simulink model "pid20180920"  (R2018b)
settings: Solver=ode3  StartTime=0.0  StopTime=5  FixedStep=0.02  RelTol=1e-3
settings Model: Creator=Think  LastModifiedBy=think
settings DataIOCC: LimitDataPoints=on  SaveFormat=Array
settings OptimizationCC: BlockReduction=off  BooleanDataType=off  LifeSpan=inf
settings DebuggingCC: SaveWithParameterizedLinksMsg=none  UnderspecifiedInitializationDetection=Classic  MergeDetectMultiDrivingBlocksExec=none  SignalResolutionControl=TryResolveAllWithWarning  SFUnexpectedBacktrackingDiag=warning  SFNoUnconditionalDefaultTransitionDiag=warning  SFExecutionAtInitializationDiag=none
settings HardwareCC: ProdBitPerPointer=32  ProdBitPerSizeT=32  ProdBitPerPtrDiffT=32  ProdLargestAtomicFloat=None  ProdIntDivRoundTo=Undefined  ProdEndianess=Unspecified  ProdWordSize=32  ProdHWDeviceType=32-bit Generic  TargetUnknown=on
settings ModelReferenceCC: PropagateSignalLabelsOutOfModel=off
settings SFSimCC: SimUseLocalCustomCode=off
settings RTWCC: RTWUseLocalCustomCode=off
settings CodeAppCC: StateflowObjectComments=on
settings GRTTargetCC: TargetLangStandard=C89/C90 (ANSI)  GeneratePreprocessorConditionals=Disable all
settings ConfigComp: CovMetricSettings=dw  CovHtmlReporting=on  CovSaveCumulativeToWorkspaceVar=on  CovSaveSingleToWorkspaceVar=on  CovExternalEMLEnable=off  CovSFcnEnable=off

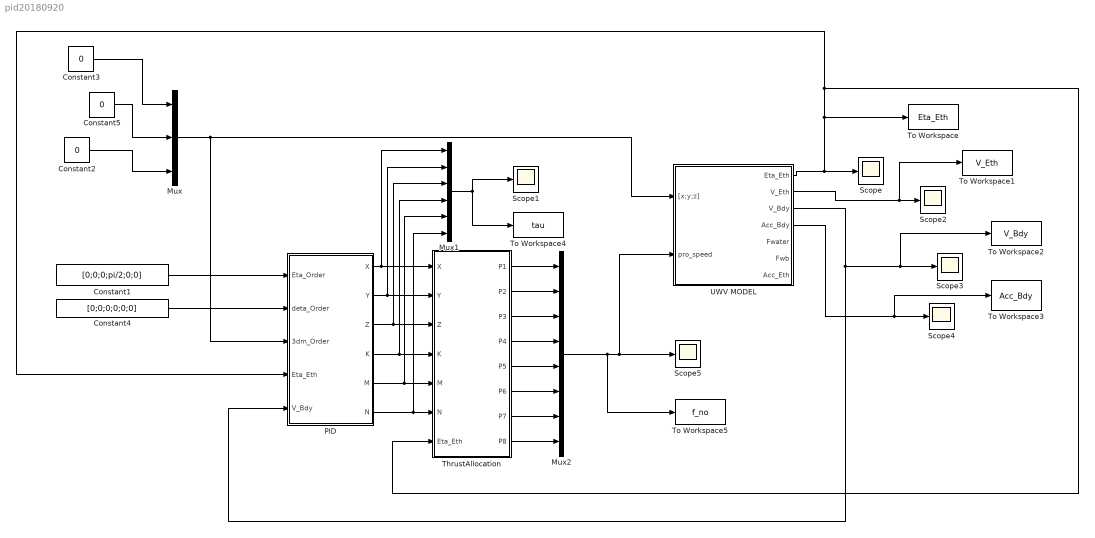
== system pid20180920 ==
  Constant1 : Constant  Value=[0;0;0;pi/2;0;0]
  Constant2 : Constant  Value=0
  Constant3 : Constant  Value=0
  Constant4 : Constant  Value=[0;0;0;0;0;0]
  Constant5 : Constant  Value=0
  Mux : Mux  Inputs=3
  Mux1 : Mux  Inputs=6
  Mux2 : Mux  Inputs=8
  PID : Subsystem
  Scope{,1..5} (6 alike) : Scope
  ThrustAllocation : Subsystem
  To Workspace : ToWorkspace  VariableName=Eta_Eth  SaveFormat=Timeseries  SampleTime=-1
  To Workspace1 : ToWorkspace  VariableName=V_Eth  SaveFormat=Timeseries  SampleTime=-1
  To Workspace2 : ToWorkspace  VariableName=V_Bdy  SaveFormat=Timeseries  SampleTime=-1
  To Workspace3 : ToWorkspace  VariableName=Acc_Bdy  SaveFormat=Timeseries  SampleTime=-1
  To Workspace4 : ToWorkspace  VariableName=tau  SaveFormat=Timeseries  SampleTime=-1
  To Workspace5 : ToWorkspace  VariableName=f_no  SaveFormat=Timeseries  SampleTime=-1
  UWV MODEL : Subsystem
  wires:
  Mux/1 -> PID/3(3dm_Order), UWV MODEL/1("[x;y;z]")
  UWV MODEL/2(V_Eth) -> To Workspace1/1, Scope2/1
  UWV MODEL/3(V_Bdy) -> PID/5(V_Bdy), To Workspace2/1, Scope3/1
  UWV MODEL/4(Acc_Bdy) -> To Workspace3/1, Scope4/1
  Constant2/1 -> Mux/3
  Constant3/1 -> Mux/1
  ThrustAllocation/1(P1) -> Mux2/1
  ThrustAllocation/2(P2) -> Mux2/2
  ThrustAllocation/3(P3) -> Mux2/3
  ThrustAllocation/4(P4) -> Mux2/4
  ThrustAllocation/5(P5) -> Mux2/5
  ThrustAllocation/6(P6) -> Mux2/6
  ThrustAllocation/7(P7) -> Mux2/7
  ThrustAllocation/8(P8) -> Mux2/8
  UWV MODEL/1(Eta_Eth) -> PID/4(Eta_Eth), ThrustAllocation/7(Eta_Eth), To Workspace/1, Scope/1
  Constant1/1 -> PID/1(Eta_Order)
  Constant4/1 -> PID/2(deta_Order)
  Mux2/1 -> To Workspace5/1, UWV MODEL/2(pro_speed), Scope5/1
  PID/1(X) -> Mux1/1, ThrustAllocation/1(X)
  PID/2(Y) -> Mux1/2, ThrustAllocation/2(Y)
  PID/3(Z) -> Mux1/3, ThrustAllocation/3(Z)
  PID/4(K) -> Mux1/4, ThrustAllocation/4(K)
  PID/5(M) -> Mux1/5, ThrustAllocation/5(M)
  PID/6(N) -> Mux1/6, ThrustAllocation/6(N)
  Mux1/1 -> To Workspace4/1, Scope1/1
  Constant5/1 -> Mux/2

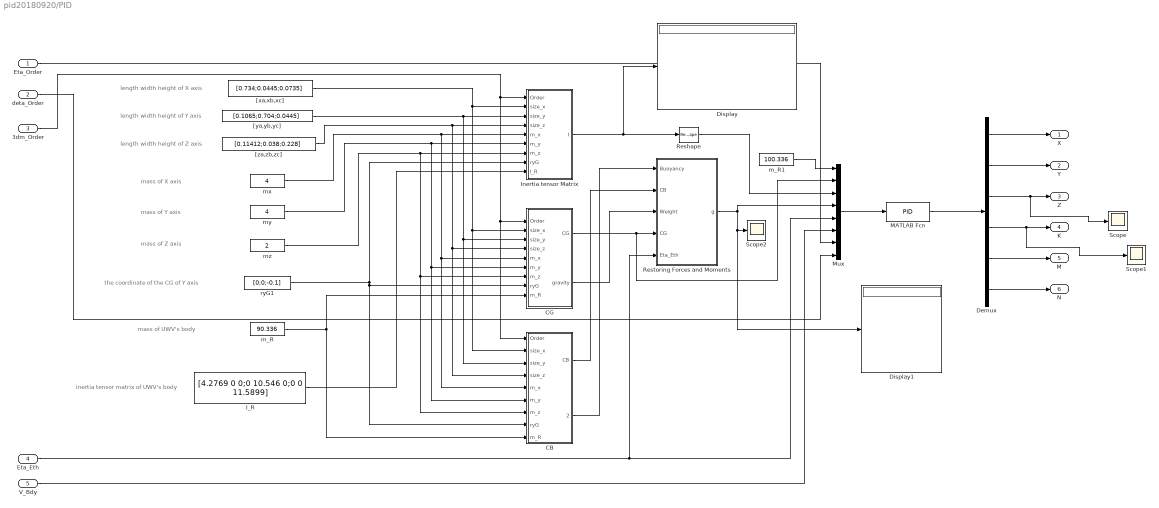
== system pid20180920/PID ==
  note: mass of Z axis
  note: mass of X axis
  note: mass of Y axis
  note: length width height of Y axis
  note: length width height of Z axis
  note: length width height of X axis
  note: the coordinate of the CG of Y axis
  note: mass of UWV's body
  note: inertia tensor matrix of UWV's body
  Eta_Order : Inport
  deta_Order : Inport  Port=2
  3dm_Order : Inport  Port=3
  Eta_Eth : Inport  Port=4
  V_Bdy : Inport  Port=5
  CB : Subsystem
  CG : Subsystem
  Demux : Demux  Outputs=6
  Display : Display
  Display1 : Display
  I_R : Constant  Value=[4.2769 0 0;0 10.546 0;0 0 11.5899]
  Inertia tensor Matrix : Subsystem
  MATLAB Fcn : MATLABFcn  MATLABFcn=PID  OutputDimensions=6  Output1D=off
  Mux : Mux  Inputs=8
  Reshape : Reshape
  Restoring Forces and Moments : Subsystem
  Scope : Scope
  Scope1 : Scope
  Scope2 : Scope
  "[xa,xb,xc]" : Constant  Value=[0.734;0.0445;0.0735]
  "[ya,yb,yc]" : Constant  Value=[0.1065;0.704;0.0445]
  "[za,zb,zc]" : Constant  Value=[0.11412;0.038;0.228]
  m_R : Constant  Value=90.336
  m_R1 : Constant  Value=100.336
  mx : Constant  Value=4
  my : Constant  Value=4
  mz : Constant  Value=2
  ryG1 : Constant  Value=[0;0;-0.1]
  X : Outport
  Y : Outport  Port=2
  Z : Outport  Port=3
  K : Outport  Port=4
  M : Outport  Port=5
  N : Outport  Port=6
  wires:
  CG/1(CG) -> Mux/2, Restoring Forces and Moments/4(CG)
  CG/2(gravity) -> Restoring Forces and Moments/3(Weight)
  CB/1(CB) -> Restoring Forces and Moments/2(CB)
  CB/2(Buoyancy) -> Restoring Forces and Moments/1(Buoyancy)
  Mux/1 -> MATLAB Fcn/1
  Reshape/1 -> Mux/3
  Eta_Eth/1 -> Restoring Forces and Moments/5(Eta_Eth), Mux/5
  V_Bdy/1 -> Mux/6
  Eta_Order/1 -> Mux/7
  "[xa,xb,xc]"/1 -> CB/2(size_x), CG/2(size_x), Inertia tensor Matrix/2(size_x)
  "[ya,yb,yc]"/1 -> CB/3(size_y), CG/3(size_y), Inertia tensor Matrix/3(size_y)
  "[za,zb,zc]"/1 -> CB/4(size_z), CG/4(size_z), Inertia tensor Matrix/4(size_z)
  mx/1 -> CB/5(m_x), CG/5(m_x), Inertia tensor Matrix/5(m_x)
  my/1 -> CB/6(m_y), CG/6(m_y), Inertia tensor Matrix/6(m_y)
  mz/1 -> CB/7(m_z), CG/7(m_z), Inertia tensor Matrix/7(m_z)
  ryG1/1 -> CB/8(ryG), CG/8(ryG), Inertia tensor Matrix/8(ryG)
  m_R/1 -> CG/9(m_R), CB/9(m_R)
  I_R/1 -> Inertia tensor Matrix/9(I_R)
  m_R1/1 -> Mux/1
  MATLAB Fcn/1 -> Demux/1
  Demux/1 -> X/1
  Demux/2 -> Y/1
  Demux/3 -> Scope/1, Z/1
  Demux/4 -> Scope1/1, K/1
  Demux/5 -> M/1
  Demux/6 -> N/1
  deta_Order/1 -> Mux/8
  Inertia tensor Matrix/1(I) -> Display/1, Reshape/1
  3dm_Order/1 -> CB/1(Order), CG/1(Order), Inertia tensor Matrix/1(Order)
  Restoring Forces and Moments/1(g) -> Scope2/1, Display1/1, Mux/4

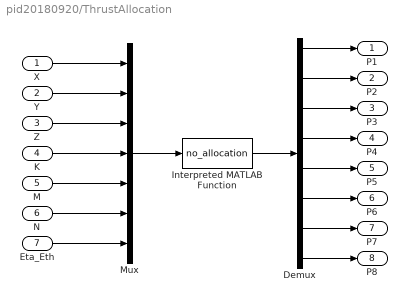
== system pid20180920/ThrustAllocation ==
  X : Inport
  Y : Inport  Port=2
  Z : Inport  Port=3
  K : Inport  Port=4
  M : Inport  Port=5
  N : Inport  Port=6
  Eta_Eth : Inport  Port=7
  Demux : Demux  Outputs=8
  Interpreted MATLAB Function : MATLABFcn  MATLABFcn=no_allocation  OutputDimensions=8
  Mux : Mux  Inputs=7
  P1 : Outport
  P2 : Outport  Port=2
  P3 : Outport  Port=3
  P4 : Outport  Port=4
  P5 : Outport  Port=5
  P6 : Outport  Port=6
  P7 : Outport  Port=7
  P8 : Outport  Port=8
  wires:
  Mux/1 -> Interpreted MATLAB Function/1
  X/1 -> Mux/1
  Y/1 -> Mux/2
  Z/1 -> Mux/3
  K/1 -> Mux/4
  M/1 -> Mux/5
  N/1 -> Mux/6
  Eta_Eth/1 -> Mux/7
  Interpreted MATLAB Function/1 -> Demux/1
  Demux/8 -> P8/1
  Demux/1 -> P1/1
  Demux/2 -> P2/1
  Demux/3 -> P3/1
  Demux/4 -> P4/1
  Demux/5 -> P5/1
  Demux/6 -> P6/1
  Demux/7 -> P7/1

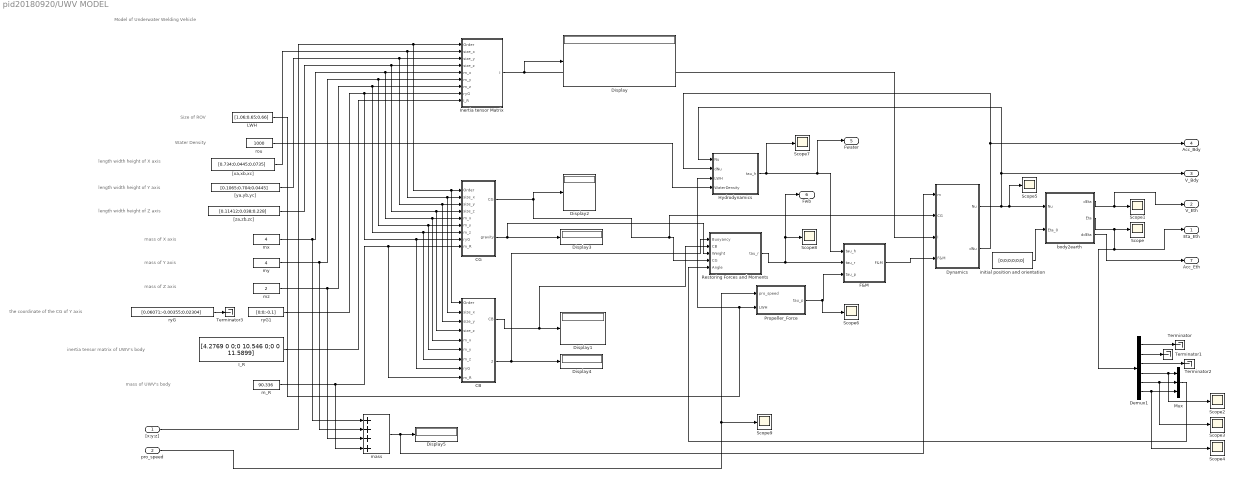
== system pid20180920/UWV MODEL ==
  note: mass of Z axis
  note: length width height of Y axis
  note: the coordinate of the CG of Y axis
  note: length width height of Z axis
  note: mass of UWV's body
  note: mass of X axis
  note: Water Density
  note: length width height of X axis
  note: mass of Y axis
  note: Size of ROV
  note: inertia tensor matrix of UWV's body
  note: Model of Underwater Welding Vehicle
  "[x;y;z]" : Inport
  pro_speed : Inport  Port=2
  CB : Subsystem
  CG : Subsystem
  Demux1 : Demux  Outputs=6
  Display{,1..5} (6 alike) : Display
  Dynamics : Subsystem
  F&M : Subsystem
  Hydrodynamics : Subsystem
  I_R : Constant  Value=[4.2769 0 0;0 10.546 0;0 0 11.5899]
  Inertia tensor Matrix : Subsystem
  LWH : Constant  Value=[1.06;0.65;0.66]
  Mux : Mux  Inputs=3
  Propeller_Force : Subsystem
  Restoring Forces and Moments : Subsystem
  Scope{,1..9} (10 alike) : Scope
  Terminator{,1..3} (4 alike) : Terminator
  "[xa,xb,xc]" : Constant  Value=[0.734;0.0445;0.0735]
  "[ya,yb,yc]" : Constant  Value=[0.1065;0.704;0.0445]
  "[za,zb,zc]" : Constant  Value=[0.11412;0.038;0.228]
  "body2earth " : Subsystem
  initial position and orientation : Constant  Value=[0;0;0;0;0;0]
  m_R : Constant  Value=90.336
  mass : Sum  Inputs=++++
      mask Display:
      | port_label('input',1,'m_x')
      | port_label('input',2,'m_y')
      | port_label('input',3,'m_z')
      | port_label('input',4,'m_R')
      | port_label('output',1,'m')
  mx : Constant  Value=4
  my : Constant  Value=4
  mz : Constant  Value=2
  rou : Constant  Value=1000
  ryG : Constant  Value=[0.06071;-0.00355;0.02304]
  ryG1 : Constant  Value=[0;0;-0.1]
  Eta_Eth : Outport
  V_Eth : Outport  Port=2
  V_Bdy : Outport  Port=3
  Acc_Bdy : Outport  Port=4
  Fwater : Outport  Port=5
  Fwb : Outport  Port=6
  Acc_Eth : Outport  Port=7
  wires:
  Dynamics/2(dNu) -> Acc_Bdy/1, Hydrodynamics/2(dNu)
  rou/1 -> Hydrodynamics/4(WaterDensity)
  mass/1 -> Dynamics/1(m), Display5/1
  Inertia tensor Matrix/1(I) -> Dynamics/3(I), Display/1
  F&M/1(F&M) -> Dynamics/4(F&M)
  Dynamics/1(Nu) -> V_Bdy/1, Hydrodynamics/1(Nu), Scope5/1, "body2earth "/1(Nu)
  initial position and orientation/1 -> "body2earth "/2(Eta_0)
  "[xa,xb,xc]"/1 -> Inertia tensor Matrix/2(size_x), CB/2(size_x), CG/2(size_x)
  m_R/1 -> mass/4, CB/9(m_R), CG/9(m_R)
  mz/1 -> mass/3, CB/7(m_z), CG/7(m_z), Inertia tensor Matrix/7(m_z)
  mx/1 -> mass/1, CB/5(m_x), CG/5(m_x), Inertia tensor Matrix/5(m_x)
  I_R/1 -> Inertia tensor Matrix/9(I_R)
  my/1 -> mass/2, CB/6(m_y), CG/6(m_y), Inertia tensor Matrix/6(m_y)
  "[ya,yb,yc]"/1 -> CB/3(size_y), CG/3(size_y), Inertia tensor Matrix/3(size_y)
  "[x;y;z]"/1 -> Inertia tensor Matrix/1(Order), CB/1(Order), CG/1(Order)
  ryG1/1 -> CB/8(ryG), CG/8(ryG), Inertia tensor Matrix/8(ryG)
  "[za,zb,zc]"/1 -> CB/4(size_z), CG/4(size_z), Inertia tensor Matrix/4(size_z)
  "body2earth "/1(dEta) -> V_Eth/1, Scope1/1
  Restoring Forces and Moments/1(tau_r) -> Fwb/1, Scope8/1, F&M/2(tau_r)
  LWH/1 -> Hydrodynamics/3(LWH), Propeller_Force/2(LWH)
  Demux1/2 -> Terminator1/1
  Demux1/4 -> Scope2/1, Mux/1
  "body2earth "/2(Eta) -> Eta_Eth/1, Demux1/1, Scope/1
  Demux1/1 -> Terminator/1
  Demux1/6 -> Scope4/1, Mux/3
  Demux1/3 -> Terminator2/1
  Demux1/5 -> Scope3/1, Mux/2
  Propeller_Force/1(tau_p) -> Scope6/1, F&M/3(tau_p)
  CG/2(gravity) -> Restoring Forces and Moments/3(Weight), Display3/1
  CB/2(Buoyancy) -> Restoring Forces and Moments/1(Buoyancy), Display4/1
  CG/1(CG) -> Dynamics/2(CG), Restoring Forces and Moments/4(CG), Display2/1
  Mux/1 -> Restoring Forces and Moments/5(Angle)
  ryG/1 -> Terminator3/1
  pro_speed/1 -> Scope9/1, Propeller_Force/1(pro_speed)
  CB/1(CB) -> Restoring Forces and Moments/2(CB), Display1/1
  Hydrodynamics/1(tau_h) -> F&M/1(tau_h), Fwater/1, Scope7/1
  "body2earth "/3(ddEta) -> Acc_Eth/1

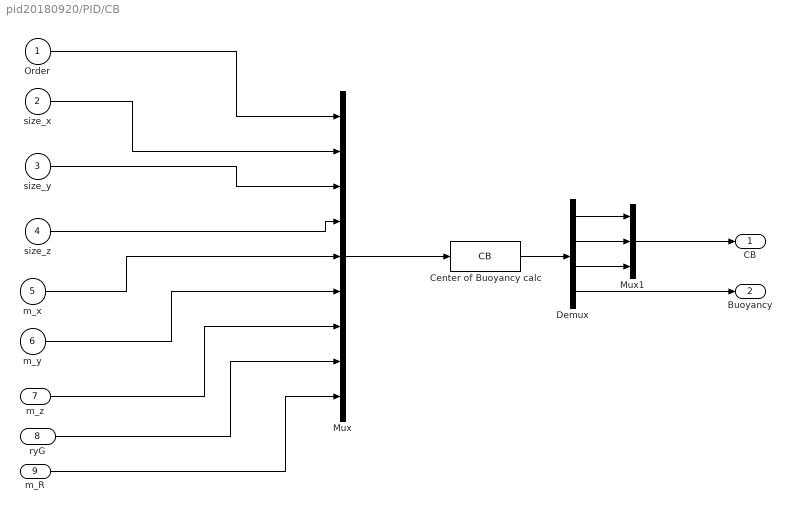
== system pid20180920/PID/CB ==
  Order : Inport
  size_x : Inport  Port=2
  size_y : Inport  Port=3
  size_z : Inport  Port=4
  m_x : Inport  Port=5
  m_y : Inport  Port=6
  m_z : Inport  Port=7
  ryG : Inport  Port=8
  m_R : Inport  Port=9
  Center of Buoyancy calc : MATLABFcn  MATLABFcn=CB  Output1D=off
  Demux : Demux
  Mux : Mux  Inputs=9
  Mux1 : Mux  Inputs=3
  CB : Outport
  Buoyancy : Outport  Port=2
  wires:
  m_x/1 -> Mux/5
  m_y/1 -> Mux/6
  size_x/1 -> Mux/2
  ryG/1 -> Mux/8
  size_z/1 -> Mux/4
  Order/1 -> Mux/1
  size_y/1 -> Mux/3
  m_R/1 -> Mux/9
  m_z/1 -> Mux/7
  Mux/1 -> Center of Buoyancy calc/1
  Center of Buoyancy calc/1 -> Demux/1
  Demux/1 -> Mux1/1
  Demux/2 -> Mux1/2
  Demux/3 -> Mux1/3
  Demux/4 -> Buoyancy/1
  Mux1/1 -> CB/1

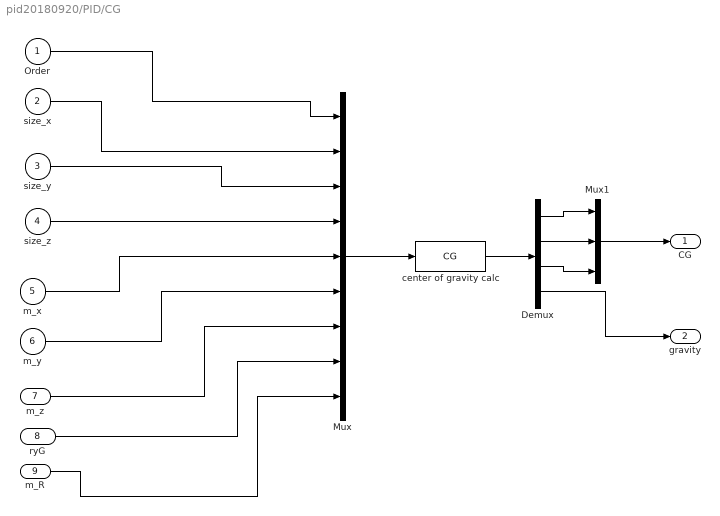
== system pid20180920/PID/CG ==
  Order : Inport
  size_x : Inport  Port=2
  size_y : Inport  Port=3
  size_z : Inport  Port=4
  m_x : Inport  Port=5
  m_y : Inport  Port=6
  m_z : Inport  Port=7
  ryG : Inport  Port=8
  m_R : Inport  Port=9
  Demux : Demux
  Mux : Mux  Inputs=9
  Mux1 : Mux  Inputs=3
  center of gravity calc : MATLABFcn  MATLABFcn=CG  Output1D=off
  CG : Outport
  gravity : Outport  Port=2
  wires:
  Mux/1 -> center of gravity calc/1
  center of gravity calc/1 -> Demux/1
  Demux/1 -> Mux1/1
  Demux/2 -> Mux1/2
  Mux1/1 -> CG/1
  Demux/4 -> gravity/1
  Order/1 -> Mux/1
  size_x/1 -> Mux/2
  size_y/1 -> Mux/3
  size_z/1 -> Mux/4
  m_x/1 -> Mux/5
  m_y/1 -> Mux/6
  ryG/1 -> Mux/8
  m_R/1 -> Mux/9
  m_z/1 -> Mux/7
  Demux/3 -> Mux1/3

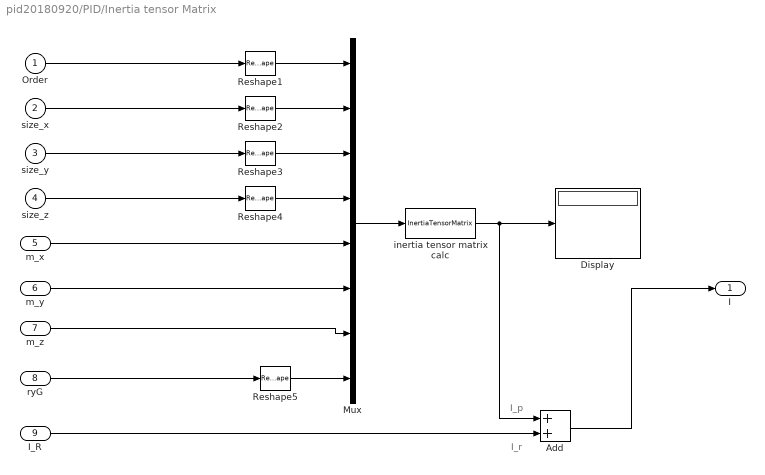
== system pid20180920/PID/Inertia tensor Matrix ==
  note: I_r
  note: I_p
  Order : Inport
  size_x : Inport  Port=2
  size_y : Inport  Port=3
  size_z : Inport  Port=4
  m_x : Inport  Port=5
  m_y : Inport  Port=6
  m_z : Inport  Port=7
  ryG : Inport  Port=8
  I_R : Inport  Port=9
  Add : Sum
  Display : Display
  Mux : Mux  Inputs=8
  Reshape{1..5} (5 alike) : Reshape  OutputDimensions=9
  inertia tensor matrix calc : MATLABFcn  MATLABFcn=InertiaTensorMatrix  Output1D=off
  I : Outport
  wires:
  inertia tensor matrix calc/1 -> Display/1, Add/1
  Mux/1 -> inertia tensor matrix calc/1
  m_z/1 -> Mux/7
  size_z/1 -> Reshape4/1
  m_x/1 -> Mux/5
  Order/1 -> Reshape1/1
  m_y/1 -> Mux/6
  size_x/1 -> Reshape2/1
  size_y/1 -> Reshape3/1
  ryG/1 -> Reshape5/1
  Add/1 -> I/1
  I_R/1 -> Add/2
  Reshape1/1 -> Mux/1
  Reshape2/1 -> Mux/2
  Reshape3/1 -> Mux/3
  Reshape4/1 -> Mux/4
  Reshape5/1 -> Mux/8

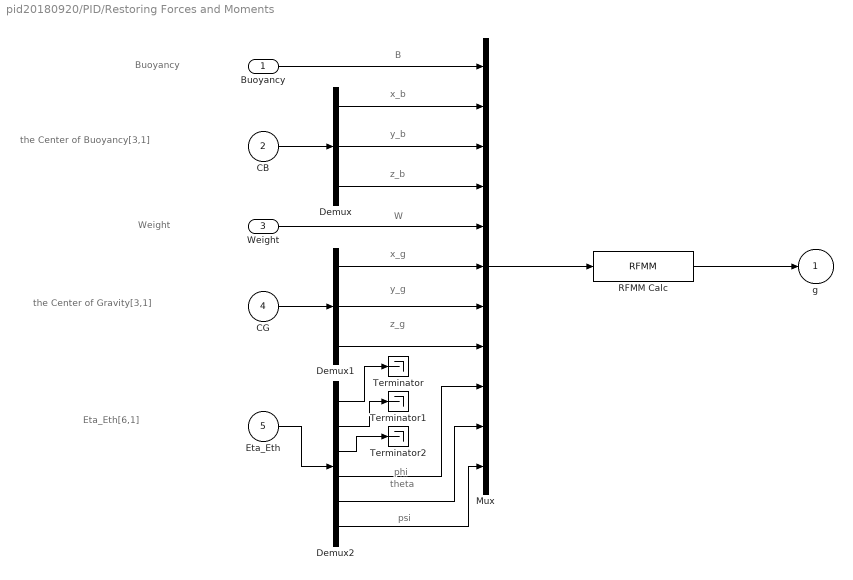
== system pid20180920/PID/Restoring Forces and Moments ==
  note: psi
  note: theta
  note: phi
  note: W
  note: x_b
  note: B
  note: Buoyancy
  note: the Center of Buoyancy[3,1]
  note: Weight
  note: the Center of Gravity[3,1]
  note: Eta_Eth[6,1]
  note: y_b
  note: z_b
  note: x_g
  note: y_g
  note: z_g
  Buoyancy : Inport
  CB : Inport  Port=2
  Weight : Inport  Port=3
  CG : Inport  Port=4
  Eta_Eth : Inport  Port=5
  Demux : Demux  Outputs=3
  Demux1 : Demux  Outputs=3
  Demux2 : Demux  Outputs=6
  Mux : Mux  Inputs=11
  RFMM Calc : MATLABFcn  MATLABFcn=RFMM  OutputDimensions=6
  Terminator : Terminator
  Terminator1 : Terminator
  Terminator2 : Terminator
  g : Outport
  wires:
  CB/1 -> Demux/1
  CG/1 -> Demux1/1
  Eta_Eth/1 -> Demux2/1
  Buoyancy/1 -> Mux/1
  Demux/1 -> Mux/2
  Demux/2 -> Mux/3
  Demux/3 -> Mux/4
  Weight/1 -> Mux/5
  Demux1/1 -> Mux/6
  Demux1/2 -> Mux/7
  Demux1/3 -> Mux/8
  Demux2/4 -> Mux/9
  Demux2/5 -> Mux/10
  Demux2/6 -> Mux/11
  Mux/1 -> RFMM Calc/1
  RFMM Calc/1 -> g/1
  Demux2/1 -> Terminator/1
  Demux2/2 -> Terminator1/1
  Demux2/3 -> Terminator2/1

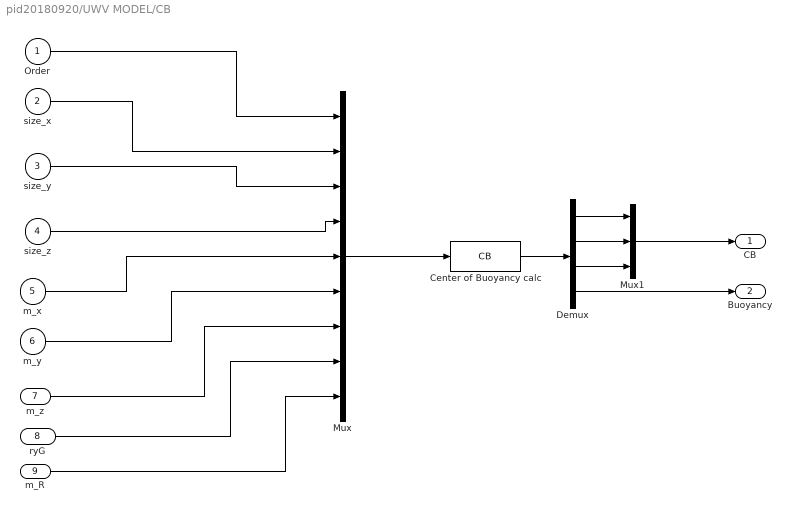
== system pid20180920/UWV MODEL/CB ==
  Order : Inport
  size_x : Inport  Port=2
  size_y : Inport  Port=3
  size_z : Inport  Port=4
  m_x : Inport  Port=5
  m_y : Inport  Port=6
  m_z : Inport  Port=7
  ryG : Inport  Port=8
  m_R : Inport  Port=9
  Center of Buoyancy calc : MATLABFcn  MATLABFcn=CB  Output1D=off
  Demux : Demux
  Mux : Mux  Inputs=9
  Mux1 : Mux  Inputs=3
  CB : Outport
  Buoyancy : Outport  Port=2
  wires:
  m_x/1 -> Mux/5
  m_y/1 -> Mux/6
  size_x/1 -> Mux/2
  ryG/1 -> Mux/8
  size_z/1 -> Mux/4
  Order/1 -> Mux/1
  size_y/1 -> Mux/3
  m_R/1 -> Mux/9
  m_z/1 -> Mux/7
  Mux/1 -> Center of Buoyancy calc/1
  Center of Buoyancy calc/1 -> Demux/1
  Demux/1 -> Mux1/1
  Demux/2 -> Mux1/2
  Demux/3 -> Mux1/3
  Demux/4 -> Buoyancy/1
  Mux1/1 -> CB/1

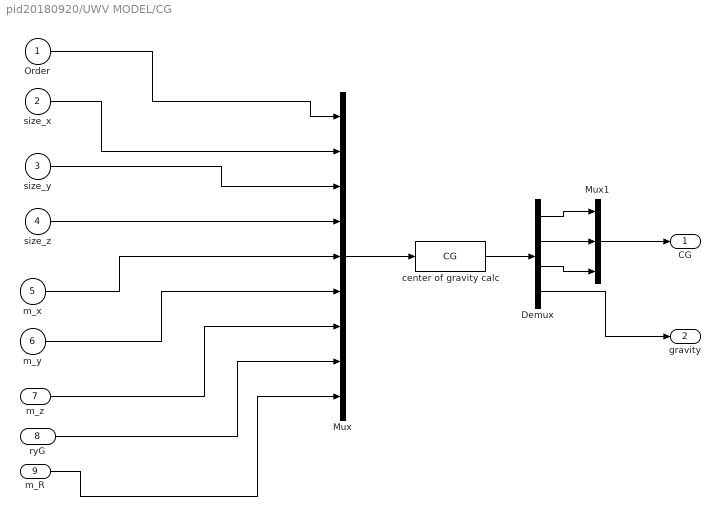
== system pid20180920/UWV MODEL/CG ==
  Order : Inport
  size_x : Inport  Port=2
  size_y : Inport  Port=3
  size_z : Inport  Port=4
  m_x : Inport  Port=5
  m_y : Inport  Port=6
  m_z : Inport  Port=7
  ryG : Inport  Port=8
  m_R : Inport  Port=9
  Demux : Demux
  Mux : Mux  Inputs=9
  Mux1 : Mux  Inputs=3
  center of gravity calc : MATLABFcn  MATLABFcn=CG  Output1D=off
  CG : Outport
  gravity : Outport  Port=2
  wires:
  Mux/1 -> center of gravity calc/1
  center of gravity calc/1 -> Demux/1
  Demux/1 -> Mux1/1
  Demux/2 -> Mux1/2
  Mux1/1 -> CG/1
  Demux/4 -> gravity/1
  Order/1 -> Mux/1
  size_x/1 -> Mux/2
  size_y/1 -> Mux/3
  size_z/1 -> Mux/4
  m_x/1 -> Mux/5
  m_y/1 -> Mux/6
  ryG/1 -> Mux/8
  m_R/1 -> Mux/9
  m_z/1 -> Mux/7
  Demux/3 -> Mux1/3

== system pid20180920/UWV MODEL/Dynamics ==
  note: velocity in earth-fix reference
  note: inertia tensor matrix
  note: tau
  note: center of gravity
  note: mass
  note: position and orientation in earth-fix reference
  m : Inport
  CG : Inport  Port=2
  I : Inport  Port=3
  F&M : Inport  Port=4
  Demux : Demux  Outputs=12
  Mux : Mux
  Mux1 : Mux  Inputs=6
  Mux2 : Mux  Inputs=6
  Reshape : Reshape
  S-Function : S-Function  FunctionName=Dynamics  SFunctionDeploymentMode=off  EnableBusSupport=off
  Nu : Outport
  dNu : Outport  Port=2
  wires:
  CG/1 -> Mux/2
  I/1 -> Reshape/1
  m/1 -> Mux/1
  Reshape/1 -> Mux/3
  F&M/1 -> Mux/4
  Mux/1 -> S-Function/1
  S-Function/1 -> Demux/1
  Demux/1 -> Mux1/1
  Demux/2 -> Mux1/2
  Demux/3 -> Mux1/3
  Demux/4 -> Mux1/4
  Demux/5 -> Mux1/5
  Demux/6 -> Mux1/6
  Mux1/1 -> Nu/1
  Demux/7 -> Mux2/1
  Demux/8 -> Mux2/2
  Demux/9 -> Mux2/3
  Demux/10 -> Mux2/4
  Demux/11 -> Mux2/5
  Demux/12 -> Mux2/6
  Mux2/1 -> dNu/1

== system pid20180920/UWV MODEL/F&M ==
  tau_h : Inport
  tau_r : Inport  Port=2
  tau_p : Inport  Port=3
  Add : Sum  Inputs=+++
  F&M : Outport
  wires:
  tau_h/1 -> Add/1
  tau_r/1 -> Add/2
  tau_p/1 -> Add/3
  Add/1 -> F&M/1

== system pid20180920/UWV MODEL/Hydrodynamics ==
  Nu : Inport
  dNu : Inport  Port=2
  LWH : Inport  Port=3
  WaterDensity : Inport  Port=4
  Demux5 : Demux  Outputs=3
  MATLAB Fcn : MATLABFcn  MATLABFcn=Hydrodynamics  OutputDimensions=6  Output1D=off
  Mux : Mux
  Saturation : Saturate  UpperLimit=0.8  LowerLimit=-0.8
  Terminator : Terminator
  Terminator1 : Terminator
  tau_h : Outport
  wires:
  MATLAB Fcn/1 -> tau_h/1
  Mux/1 -> MATLAB Fcn/1
  LWH/1 -> Demux5/1
  Demux5/2 -> Terminator/1
  Demux5/3 -> Terminator1/1
  Nu/1 -> Saturation/1
  Saturation/1 -> Mux/1
  dNu/1 -> Mux/2
  Demux5/1 -> Mux/3
  WaterDensity/1 -> Mux/4

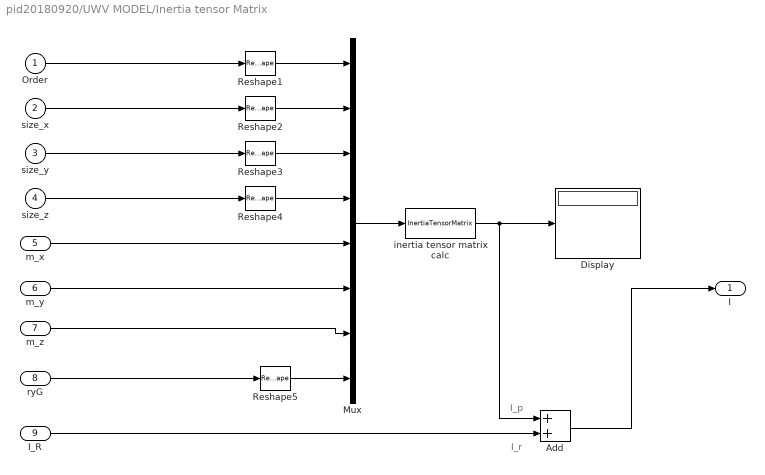
== system pid20180920/UWV MODEL/Inertia tensor Matrix ==
  note: I_r
  note: I_p
  Order : Inport
  size_x : Inport  Port=2
  size_y : Inport  Port=3
  size_z : Inport  Port=4
  m_x : Inport  Port=5
  m_y : Inport  Port=6
  m_z : Inport  Port=7
  ryG : Inport  Port=8
  I_R : Inport  Port=9
  Add : Sum
  Display : Display
  Mux : Mux  Inputs=8
  Reshape{1..5} (5 alike) : Reshape  OutputDimensions=9
  inertia tensor matrix calc : MATLABFcn  MATLABFcn=InertiaTensorMatrix  Output1D=off
  I : Outport
  wires:
  inertia tensor matrix calc/1 -> Display/1, Add/1
  Mux/1 -> inertia tensor matrix calc/1
  m_z/1 -> Mux/7
  size_z/1 -> Reshape4/1
  m_x/1 -> Mux/5
  Order/1 -> Reshape1/1
  m_y/1 -> Mux/6
  size_x/1 -> Reshape2/1
  size_y/1 -> Reshape3/1
  ryG/1 -> Reshape5/1
  Add/1 -> I/1
  I_R/1 -> Add/2
  Reshape1/1 -> Mux/1
  Reshape2/1 -> Mux/2
  Reshape3/1 -> Mux/3
  Reshape4/1 -> Mux/4
  Reshape5/1 -> Mux/8

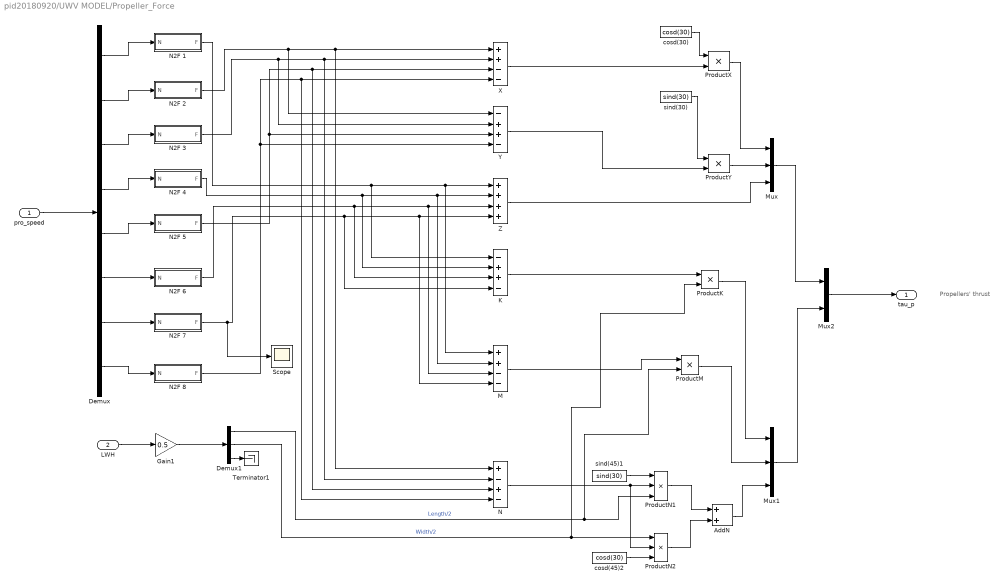
== system pid20180920/UWV MODEL/Propeller_Force ==
  note: Propellers' thrust
  pro_speed : Inport
  LWH : Inport  Port=2
  AddN : Sum
  Demux : Demux  Outputs=8
  Demux1 : Demux  Outputs=3
  Gain1 : Gain  Gain=0.5
  K : Sum  Inputs=-++-
  M : Sum  Inputs=++--
  Mux : Mux  Inputs=3
  Mux1 : Mux  Inputs=3
  Mux2 : Mux  Inputs=2
  N : Sum  Inputs=+-+-
  N2F 1 : Subsystem
  N2F 2 : Subsystem
  N2F 3 : Subsystem
  N2F 4 : Subsystem
  N2F 5 : Subsystem
  N2F 6 : Subsystem
  N2F 7 : Subsystem
  N2F 8 : Subsystem
  ProductK : Product
  ProductM : Product
  ProductN1 : Product  Inputs=3
  ProductN2 : Product  Inputs=3
  ProductX : Product
  ProductY : Product
  Scope : Scope
  Terminator1 : Terminator
  X : Sum  Inputs=++--
  Y : Sum  Inputs=-++-
  Z : Sum  Inputs=++++
  cosd(30) : Constant  Value=cosd(30)
  cosd(45)2 : Constant  Value=cosd(30)
  sind(30) : Constant  Value=sind(30)
  sind(45)1 : Constant  Value=sind(30)
  tau_p : Outport
  wires:
  Mux1/1 -> Mux2/2
  Mux/1 -> Mux2/1
  X/1 -> ProductX/2
  ProductX/1 -> Mux/1
  ProductY/1 -> Mux/2
  Y/1 -> ProductY/2
  Z/1 -> Mux/3
  Demux1/3 -> Terminator1/1
  Gain1/1 -> Demux1/1
  LWH/1 -> Gain1/1
  cosd(30)/1 -> ProductX/1
  sind(30)/1 -> ProductY/1
  N/1 -> ProductN2/2, ProductN1/2
  sind(45)1/1 -> ProductN1/1
  cosd(45)2/1 -> ProductN2/3
  Demux1/1 -> ProductM/2, ProductN1/3  "Length/2"
  Demux1/2 -> ProductN2/1, ProductK/2  "Width/2"
  ProductN1/1 -> AddN/1
  ProductN2/1 -> AddN/2
  AddN/1 -> Mux1/3
  K/1 -> ProductK/1
  M/1 -> ProductM/1
  ProductK/1 -> Mux1/1
  ProductM/1 -> Mux1/2
  Mux2/1 -> tau_p/1
  N2F 2/1(F) -> Y/1, X/1, N/1
  N2F 3/1(F) -> Y/2, X/2, N/2
  N2F 5/1(F) -> X/3, N/3, Y/3
  N2F 8/1(F) -> X/4, N/4, Y/4
  N2F 4/1(F) -> K/2, M/2, Z/2
  N2F 6/1(F) -> K/3, M/3, Z/3
  N2F 1/1(F) -> K/1, M/1, Z/1
  N2F 7/1(F) -> Scope/1, K/4, M/4, Z/4
  Demux/8 -> N2F 8/1(N)
  Demux/1 -> N2F 1/1(N)
  Demux/2 -> N2F 2/1(N)
  Demux/3 -> N2F 3/1(N)
  Demux/4 -> N2F 4/1(N)
  Demux/5 -> N2F 5/1(N)
  Demux/6 -> N2F 6/1(N)
  Demux/7 -> N2F 7/1(N)
  pro_speed/1 -> Demux/1

== system pid20180920/UWV MODEL/Restoring Forces and Moments ==
  note: psi
  note: theta
  note: phi
  note: W
  note: x_b
  note: B
  note: Buoyancy
  note: the Center of Buoyancy[3,1]
  note: Weight
  note: the Center of Gravity[3,1]
  note: orientation[3,1]
  note: y_b
  note: z_b
  note: x_g
  note: y_g
  note: z_g
  Buoyancy : Inport
  CB : Inport  Port=2
  Weight : Inport  Port=3
  CG : Inport  Port=4
  Angle : Inport  Port=5
  Demux : Demux  Outputs=3
  Demux1 : Demux  Outputs=3
  Demux2 : Demux  Outputs=3
  Mux : Mux  Inputs=11
  RFMM Calc : MATLABFcn  MATLABFcn=RFMM  OutputDimensions=6
  tau_r : Outport
  wires:
  CB/1 -> Demux/1
  CG/1 -> Demux1/1
  Angle/1 -> Demux2/1
  Buoyancy/1 -> Mux/1
  Demux/1 -> Mux/2
  Demux/2 -> Mux/3
  Demux/3 -> Mux/4
  Weight/1 -> Mux/5
  Demux1/1 -> Mux/6
  Demux1/2 -> Mux/7
  Demux1/3 -> Mux/8
  Demux2/1 -> Mux/9
  Demux2/2 -> Mux/10
  Demux2/3 -> Mux/11
  Mux/1 -> RFMM Calc/1
  RFMM Calc/1 -> tau_r/1

== system pid20180920/UWV MODEL/body2earth  ==
  note: psi
  note: theta
  note: phi
  note: z
  note: y
  note: x
  Nu : Inport
  Eta_0 : Inport  Port=2
  Add : Sum
  Demux : Demux  Outputs=6
  Derivative : Derivative
  Integrator : Integrator
  Kinematics : Subsystem
  Mux1 : Mux  Inputs=6
  Saturation : Saturate  UpperLimit=1.4  LowerLimit=-1.4
  dEta : Outport
  Eta : Outport  Port=2
  ddEta : Outport  Port=3
  wires:
  Integrator/1 -> Add/1
  Eta_0/1 -> Add/2
  Add/1 -> Demux/1
  Demux/1 -> Mux1/1
  Demux/2 -> Mux1/2
  Demux/4 -> Mux1/4
  Demux/6 -> Mux1/6
  Demux/5 -> Saturation/1
  Saturation/1 -> Mux1/5
  Mux1/1 -> Kinematics/2(Eta), Eta/1
  Kinematics/1(dEta) -> Derivative/1, dEta/1, Integrator/1
  Nu/1 -> Kinematics/1(Nu)
  Demux/3 -> Mux1/3
  Derivative/1 -> ddEta/1

== system pid20180920/UWV MODEL/Propeller_Force/N2F 1 ==
  note: N2F模块为转速与推力之间的转换，实验数据利用推力测试得出
  N : Inport
  Negative : Fcn  Expr=-1.926e-5*u^2
  Positive : Fcn  Expr=1.926e-5*u^2
  Switch : Switch  Criteria=u2 > Threshold
  F : Outport
  wires:
  N/1 -> Negative/1, Positive/1, Switch/2
  Switch/1 -> F/1
  Positive/1 -> Switch/1
  Negative/1 -> Switch/3

== system pid20180920/UWV MODEL/Propeller_Force/N2F 2 ==
  note: N2F模块为转速与推力之间的转换，实验数据利用推力测试得出
  N : Inport
  Negative : Fcn  Expr=-1.926e-5*u^2
  Positive : Fcn  Expr=1.926e-5*u^2
  Switch : Switch  Criteria=u2 > Threshold
  F : Outport
  wires:
  N/1 -> Negative/1, Positive/1, Switch/2
  Switch/1 -> F/1
  Positive/1 -> Switch/1
  Negative/1 -> Switch/3

== system pid20180920/UWV MODEL/Propeller_Force/N2F 3 ==
  note: N2F模块为转速与推力之间的转换，实验数据利用推力测试得出
  N : Inport
  Negative : Fcn  Expr=-1.926e-5*u^2
  Positive : Fcn  Expr=1.926e-5*u^2
  Switch : Switch  Criteria=u2 > Threshold
  F : Outport
  wires:
  N/1 -> Negative/1, Positive/1, Switch/2
  Switch/1 -> F/1
  Positive/1 -> Switch/1
  Negative/1 -> Switch/3

== system pid20180920/UWV MODEL/Propeller_Force/N2F 4 ==
  note: N2F模块为转速与推力之间的转换，实验数据利用推力测试得出
  N : Inport
  Negative : Fcn  Expr=-1.926e-5*u^2
  Positive : Fcn  Expr=1.926e-5*u^2
  Switch : Switch  Criteria=u2 > Threshold
  F : Outport
  wires:
  N/1 -> Negative/1, Positive/1, Switch/2
  Switch/1 -> F/1
  Positive/1 -> Switch/1
  Negative/1 -> Switch/3

== system pid20180920/UWV MODEL/Propeller_Force/N2F 5 ==
  note: N2F模块为转速与推力之间的转换，实验数据利用推力测试得出
  N : Inport
  Negative : Fcn  Expr=-1.926e-5*u^2
  Positive : Fcn  Expr=1.926e-5*u^2
  Switch : Switch  Criteria=u2 > Threshold
  F : Outport
  wires:
  N/1 -> Negative/1, Positive/1, Switch/2
  Switch/1 -> F/1
  Positive/1 -> Switch/1
  Negative/1 -> Switch/3

== system pid20180920/UWV MODEL/Propeller_Force/N2F 6 ==
  note: N2F模块为转速与推力之间的转换，实验数据利用推力测试得出
  N : Inport
  Negative : Fcn  Expr=-1.926e-5*u^2
  Positive : Fcn  Expr=1.926e-5*u^2
  Switch : Switch  Criteria=u2 > Threshold
  F : Outport
  wires:
  N/1 -> Negative/1, Positive/1, Switch/2
  Switch/1 -> F/1
  Positive/1 -> Switch/1
  Negative/1 -> Switch/3

== system pid20180920/UWV MODEL/Propeller_Force/N2F 7 ==
  note: N2F模块为转速与推力之间的转换，实验数据利用推力测试得出
  N : Inport
  Negative : Fcn  Expr=-1.926e-5*u^2
  Positive : Fcn  Expr=1.926e-5*u^2
  Switch : Switch  Criteria=u2 > Threshold
  F : Outport
  wires:
  N/1 -> Negative/1, Positive/1, Switch/2
  Switch/1 -> F/1
  Positive/1 -> Switch/1
  Negative/1 -> Switch/3

== system pid20180920/UWV MODEL/Propeller_Force/N2F 8 ==
  note: N2F模块为转速与推力之间的转换，实验数据利用推力测试得出
  N : Inport
  Negative : Fcn  Expr=-1.926e-5*u^2
  Positive : Fcn  Expr=1.926e-5*u^2
  Switch : Switch  Criteria=u2 > Threshold
  F : Outport
  wires:
  N/1 -> Negative/1, Positive/1, Switch/2
  Switch/1 -> F/1
  Positive/1 -> Switch/1
  Negative/1 -> Switch/3

== system pid20180920/UWV MODEL/body2earth /Kinematics ==
  Nu : Inport
  Eta : Inport  Port=2
  Kinematics Calc : MATLABFcn  MATLABFcn=Kinematics
  Mux : Mux  Inputs=2
  dEta : Outport
  wires:
  Kinematics Calc/1 -> dEta/1
  Nu/1 -> Mux/1
  Mux/1 -> Kinematics Calc/1
  Eta/1 -> Mux/2
